simulink model "Calculatrice"  (R2016b)
settings: Solver=VariableStepAuto  StartTime=0.0  StopTime=10.0  RelTol=1e-3
libraries: commutil2 x3
settings Model: Creator=rcostado  LastModifiedBy=rcostado

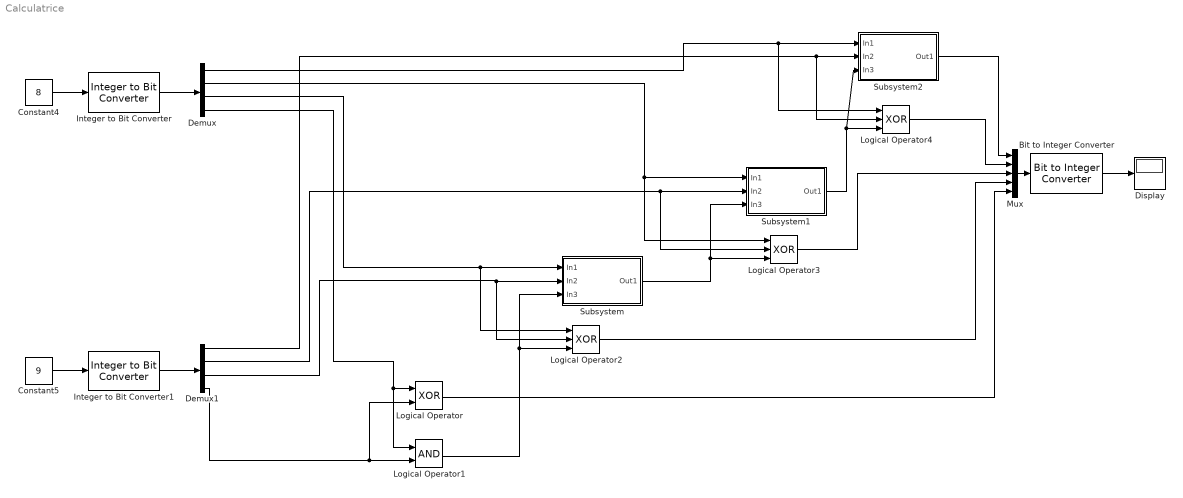
== system Calculatrice ==
  Bit to Integer Converter : commutil2/Bit to Integer Converter  nbits=5  bitOrder=MSB first  signedOutputValues=Unsigned  outDtype=Inherit via internal rule  outDtypeSigned=Inherit via internal rule
  Constant4 : Constant  Value=8
  Constant5 : Constant  Value=9
  Demux : Demux
  Demux1 : Demux
  Display : Display
  Integer to Bit Converter : commutil2/Integer to Bit Converter  nbits=4  signedInputValues=Unsigned  bitOrder=MSB first  outDtype=Inherit via internal rule
  Integer to Bit Converter1 : commutil2/Integer to Bit Converter  nbits=4  signedInputValues=Unsigned  bitOrder=MSB first  outDtype=Inherit via internal rule
  Logical Operator : Logic  Operator=XOR  AllPortsSameDT=off  OutDataTypeStr=boolean
  Logical Operator1 : Logic  AllPortsSameDT=off  OutDataTypeStr=boolean
  Logical Operator2 : Logic  Operator=XOR  Inputs=3  AllPortsSameDT=off  OutDataTypeStr=boolean
  Logical Operator3 : Logic  Operator=XOR  Inputs=3  AllPortsSameDT=off  OutDataTypeStr=boolean
  Logical Operator4 : Logic  Operator=XOR  Inputs=3  AllPortsSameDT=off  OutDataTypeStr=boolean
  Mux : Mux  Inputs=5
  Subsystem : Subsystem
  Subsystem1 : Subsystem
  Subsystem2 : Subsystem
  wires:
  Mux/1 -> Bit to Integer Converter/1
  Bit to Integer Converter/1 -> Display/1
  Integer to Bit Converter1/1 -> Demux1/1
  Constant5/1 -> Integer to Bit Converter1/1
  Constant4/1 -> Integer to Bit Converter/1
  Integer to Bit Converter/1 -> Demux/1
  Demux/4 -> Logical Operator1/1, Logical Operator/1
  Demux1/4 -> Logical Operator1/2, Logical Operator/2
  Logical Operator/1 -> Mux/5
  Logical Operator1/1 -> Subsystem/3(In3), Logical Operator2/3
  Demux1/3 -> Logical Operator2/2, Subsystem/2(In2)
  Demux/3 -> Subsystem/1(In1), Logical Operator2/1
  Logical Operator2/1 -> Mux/4
  Subsystem/1(Out1) -> Subsystem1/3(In3), Logical Operator3/3
  Demux1/2 -> Logical Operator3/2, Subsystem1/2(In2)
  Demux/2 -> Logical Operator3/1, Subsystem1/1(In1)
  Logical Operator3/1 -> Mux/3
  Subsystem1/1(Out1) -> Logical Operator4/3, Subsystem2/3(In3)
  Demux1/1 -> Subsystem2/2(In2), Logical Operator4/2
  Demux/1 -> Subsystem2/1(In1), Logical Operator4/1
  Subsystem2/1(Out1) -> Mux/1
  Logical Operator4/1 -> Mux/2

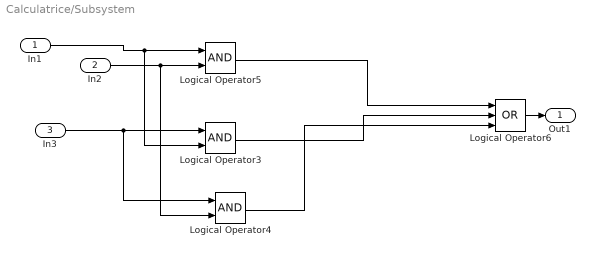
== system Calculatrice/Subsystem ==
  In1 : Inport
  In2 : Inport  Port=2
  In3 : Inport  Port=3
  Logical Operator3 : Logic  AllPortsSameDT=off  OutDataTypeStr=boolean
  Logical Operator4 : Logic  AllPortsSameDT=off  OutDataTypeStr=boolean
  Logical Operator5 : Logic  AllPortsSameDT=off  OutDataTypeStr=boolean
  Logical Operator6 : Logic  Operator=OR  Inputs=3  AllPortsSameDT=off  OutDataTypeStr=boolean
  Out1 : Outport
  wires:
  Logical Operator6/1 -> Out1/1
  Logical Operator5/1 -> Logical Operator6/1
  In3/1 -> Logical Operator4/1, Logical Operator3/1
  In2/1 -> Logical Operator4/2, Logical Operator5/2
  Logical Operator3/1 -> Logical Operator6/2
  In1/1 -> Logical Operator3/2, Logical Operator5/1
  Logical Operator4/1 -> Logical Operator6/3

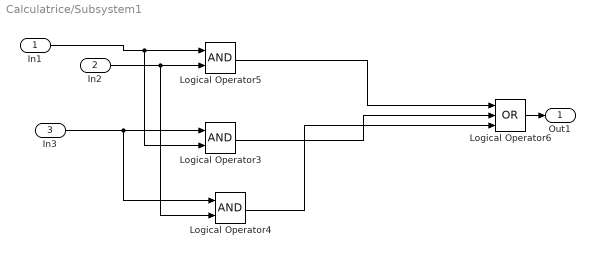
== system Calculatrice/Subsystem1 ==
  In1 : Inport
  In2 : Inport  Port=2
  In3 : Inport  Port=3
  Logical Operator3 : Logic  AllPortsSameDT=off  OutDataTypeStr=boolean
  Logical Operator4 : Logic  AllPortsSameDT=off  OutDataTypeStr=boolean
  Logical Operator5 : Logic  AllPortsSameDT=off  OutDataTypeStr=boolean
  Logical Operator6 : Logic  Operator=OR  Inputs=3  AllPortsSameDT=off  OutDataTypeStr=boolean
  Out1 : Outport
  wires:
  Logical Operator6/1 -> Out1/1
  Logical Operator5/1 -> Logical Operator6/1
  In3/1 -> Logical Operator4/1, Logical Operator3/1
  In2/1 -> Logical Operator4/2, Logical Operator5/2
  Logical Operator3/1 -> Logical Operator6/2
  In1/1 -> Logical Operator3/2, Logical Operator5/1
  Logical Operator4/1 -> Logical Operator6/3

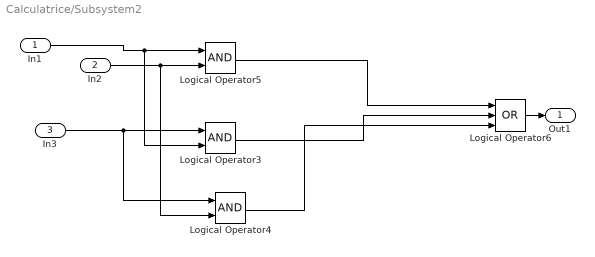
== system Calculatrice/Subsystem2 ==
  In1 : Inport
  In2 : Inport  Port=2
  In3 : Inport  Port=3
  Logical Operator3 : Logic  AllPortsSameDT=off  OutDataTypeStr=boolean
  Logical Operator4 : Logic  AllPortsSameDT=off  OutDataTypeStr=boolean
  Logical Operator5 : Logic  AllPortsSameDT=off  OutDataTypeStr=boolean
  Logical Operator6 : Logic  Operator=OR  Inputs=3  AllPortsSameDT=off  OutDataTypeStr=boolean
  Out1 : Outport
  wires:
  Logical Operator6/1 -> Out1/1
  Logical Operator5/1 -> Logical Operator6/1
  In3/1 -> Logical Operator4/1, Logical Operator3/1
  In2/1 -> Logical Operator4/2, Logical Operator5/2
  Logical Operator3/1 -> Logical Operator6/2
  In1/1 -> Logical Operator3/2, Logical Operator5/1
  Logical Operator4/1 -> Logical Operator6/3
